simulink model "es_VI_2_1"  (Simulink 8.3)
settings: Solver=ode45  StartTime=0.0  StopTime=200.0  RelTol=1e-5
values from neighbouring files (symbols this model uses):
  Kc = -0.1    [es_VI_2.m]
  Kr = 0.5    [es_VI_2.m]
libraries: cstblocks x1, simulink x1
settings Model: Creator=Indri  LastModifiedBy=Indri  ExtModeTrigMode=oneshot  ExtModeArmWhenConnect=off
settings DataIOCC: LimitDataPoints=off
settings OptimizationCC: BlockReduction=off  BooleanDataType=off  ExpressionDepthLimit=2147483647  InitFltsAndDblsToZero=on
settings DebuggingCC: SaveWithParameterizedLinksMsg=none  SignalResolutionControl=TryResolveAllWithWarning  SolverPrmCheckMsg=none  MultiTaskDSMMsg=warning  MultiTaskCondExecSysMsg=none  FcnCallInpInsideContextMsg=UseLocalSettings
settings HardwareCC: TargetUnknown=on
settings RTWCC: IncludeERTFirstTime=on

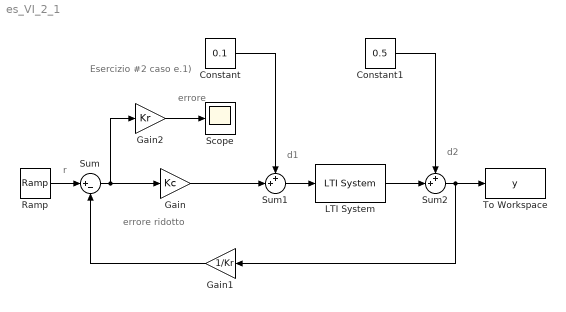
== system es_VI_2_1 ==
  note: errore
      | ridotto
  note: errore
  note: Esercizio #2
      | caso e.1)
  note: r
  note: d1
  note: d2
  Constant : Constant  Value=0.1
  Constant1 : Constant  Value=0.5
  Gain : Gain  Gain=Kc  SaturateOnIntegerOverflow=on  OutDataTypeStr=Inherit: Same as input  ParamDataTypeStr=Inherit: Same as input
  Gain1 : Gain  Gain=1/Kr  SaturateOnIntegerOverflow=on  OutDataTypeStr=Inherit: Same as input  ParamDataTypeStr=Inherit: Same as input
  Gain2 : Gain  Gain=Kr  SaturateOnIntegerOverflow=on  OutDataTypeStr=Inherit: Same as input  ParamDataTypeStr=Inherit: Same as input
  LTI System : cstblocks/LTI System  sys=F  IC=[]
  Ramp : simulink/Sources/Ramp  slope=1  start=0  X0=0
  Scope : Scope
  Sum : Sum  Inputs=|+-  SaturateOnIntegerOverflow=on  InputSameDT=on  OutDataTypeStr=Inherit: Same as first input
  Sum1 : Sum  Inputs=++|  SaturateOnIntegerOverflow=on  InputSameDT=on  OutDataTypeStr=Inherit: Same as first input
  Sum2 : Sum  Inputs=++|  SaturateOnIntegerOverflow=on  InputSameDT=on  OutDataTypeStr=Inherit: Same as first input
  To Workspace : ToWorkspace  VariableName=y  SampleTime=-1
  wires:
  Ramp/1 -> Sum/1
  Gain/1 -> Sum1/2
  Gain1/1 -> Sum/2
  Sum/1 -> Gain/1, Gain2/1
  Gain2/1 -> Scope/1
  Constant/1 -> Sum1/1
  Sum1/1 -> LTI System/1
  LTI System/1 -> Sum2/2
  Constant1/1 -> Sum2/1
  Sum2/1 -> To Workspace/1, Gain1/1
